simulink model "MC_PB_ESS3"  (Simulink 3.00)
settings: Solver=ode1  SolverMode=SingleTasking  StartTime=0.0  StopTime=2  FixedStep=1  RelTol=1e-3  AbsTol=1e-6
values from neighbouring files (symbols this model uses):
  ess_init_soc = vinf.test.ess_init_soc.FUDS    [J17_FUDS.m]    (also in J17_HFEDS.m = vinf.test.ess_init_soc.HWFET; J17_SC03.m = vinf.test.ess_init_soc.SC03; J17_UDDS.m = vinf.test.ess_init_soc.UDDS; J17_US06.m = vinf.test.ess_init_soc.US06)
undefined symbols (not defined in the file or in its folder): acc_elec_eff, acc_elec_pwr, ess_coulombic_eff, ess_max_ah_cap, ess_max_volts, ess_min_volts, ess_module_num, ess_on, ess_soc_current, ess_tmp, mc_inertia, mc_inpwr_map, mc_map_spd, mc_map_trq, mc_max_crrnt, mc_max_trq, mc_min_volts, mc_overtrq_factor, mc_spd_scale, mc_trq_scale, Tess, Tm, wm
settings Model: LastModifiedBy=vjohnson

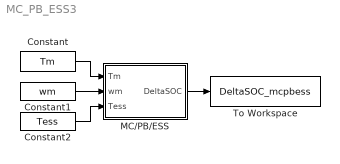
== system MC_PB_ESS3 ==
  Constant : Constant  Value=Tm
  Constant1 : Constant  Value=wm
  Constant2 : Constant  Value=Tess
  MC/PB/ESS : Subsystem
  To Workspace : ToWorkspace  VariableName=DeltaSOC_mcpbess  SampleTime=-1  SaveFormat=Matrix
  wires:
  Constant/1 -> MC/PB/ESS/1(Tm)
  Constant1/1 -> MC/PB/ESS/2(wm)
  MC/PB/ESS/1(DeltaSOC) -> To Workspace/1
  Constant2/1 -> MC/PB/ESS/3(Tess)

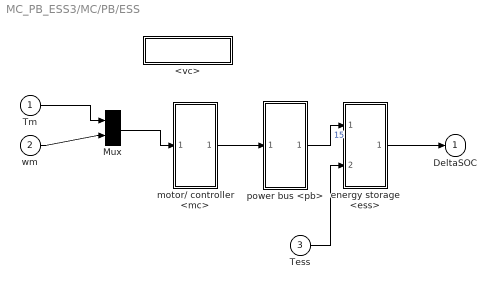
== system MC_PB_ESS3/MC/PB/ESS ==
  Tm : Inport  Port=1  PortWidth=-1  SampleTime=-1  DataType=auto
      settings: SignalType=auto
  wm : Inport  Port=2  PortWidth=-1  SampleTime=-1  DataType=auto
      settings: SignalType=auto
  Tess : Inport  Port=3  PortWidth=-1  SampleTime=-1  DataType=auto
      settings: SignalType=auto
  <vc> : Subsystem
      mask Display: disp('vehicle controls')
  Mux : Mux  Inputs=2
      settings: DisplayOption=none
  energy storage <ess> : Subsystem
  motor/ controller <mc> : Subsystem
  power bus <pb> : Subsystem
  DeltaSOC : Outport  Port=1  InitialOutput=0
  wires:
  Tm/1 -> Mux/1
  wm/1 -> Mux/2
  Mux/1 -> motor/ controller <mc>/1("torque and speed  req'd at rotor (Nm), (rad/s)")
  energy storage <ess>/1(delta SOC) -> DeltaSOC/1
  Tess/1 -> energy storage <ess>/2(Tess)
  power bus <pb>/1(power req'd from energy storage (W)) -> energy storage <ess>/1(power req'd into bus (W))  "15"
  motor/ controller <mc>/1(req'd motor input power (W)) -> power bus <pb>/1(req'd power output (W))

== system MC_PB_ESS3/MC/PB/ESS/<vc> ==
  motor controller logic : Subsystem
  shifting : Constant  Orientation=left  Value=0
  tag scope: P_mc_in_r=global
  wires:
  motor controller logic/1(req'd input power (W)1) -> [P_mc_in_r]
  [w_mc_out_r] -> motor controller logic/3(req'd output spd (rad/s))
  [P_mc_in_1lim] -> motor controller logic/2(req'd input power (W))
  [bus_voltage] -> motor controller logic/1(bus voltage)
  shifting/1 -> motor controller logic/4(shifting)

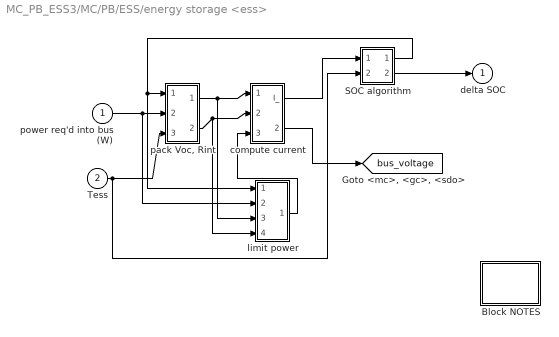
== system MC_PB_ESS3/MC/PB/ESS/energy storage <ess> ==
  power req'd into bus (W) : Inport  Port=1  PortWidth=-1  SampleTime=-1  DataType=auto
      settings: SignalType=auto
  Tess : Inport  Port=2  PortWidth=-1  SampleTime=-1  DataType=auto
      settings: SignalType=auto
  Block NOTES : Subsystem
      mask Display: disp('Block\nNOTES')
  SOC algorithm : Subsystem
  compute current : Subsystem
  limit power : Subsystem
  "pack Voc, Rint" : Subsystem
  delta SOC : Outport  Port=1  InitialOutput=0
  tag scope: bus_voltage=global
  wires:
  "pack Voc, Rint"/2(pack resistance) -> compute current/2(Rint), limit power/4(Rint)
  "pack Voc, Rint"/1(pack open- circuit voltage) -> compute current/1(Voc), limit power/3(Voc)
  SOC algorithm/1(SOC1) -> "pack Voc, Rint"/1(SOC (prev)), limit power/1(SOC)
  Tess/1 -> "pack Voc, Rint"/3(mod tmp   (C)), SOC algorithm/2(tmp (C))
  power req'd into bus (W)/1 -> "pack Voc, Rint"/2(req'd battery power (W)), limit power/2(Pbty)
  SOC algorithm/2(DeltaSOC) -> delta SOC/1
  compute current/2(V_) -> [bus_voltage]
  compute current/1(I_) -> SOC algorithm/1((A))
  limit power/1("Pbty, limited") -> compute current/3(limited output power (W))

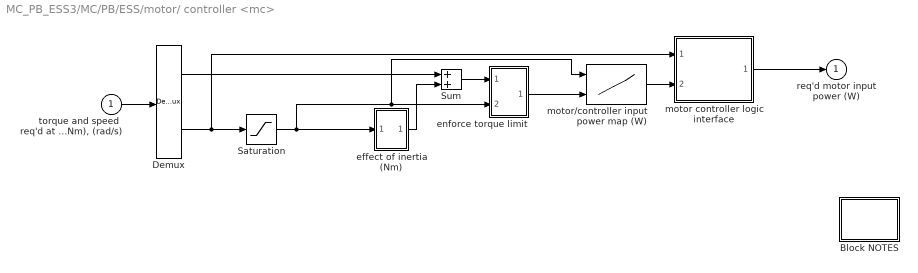
== system MC_PB_ESS3/MC/PB/ESS/motor/ controller <mc> ==
  "torque and speed  req'd at rotor (Nm), (rad/s)" : Inport  Port=1  PortWidth=-1  SampleTime=-1  DataType=auto
      settings: SignalType=auto
  Block NOTES : Subsystem
      mask Display: disp('Block\nNOTES')
  Demux : Demux  Outputs=2
  Saturation : Saturate  UpperLimit=max(mc_map_spd)*mc_spd_scale  LowerLimit=0
  Sum : Sum  Inputs=++  SaturateOnIntegerOverflow=on
  effect of inertia (Nm) : Subsystem
  enforce torque limit : Subsystem
  motor controller logic interface : Subsystem
  motor/controller input power map (W) : Lookup2D  RowIndex=mc_map_spd*mc_spd_scale  ColumnIndex=mc_map_trq*mc_trq_scale  OutputValues=mc_inpwr_map*mc_spd_scale*mc_trq_scale
  req'd motor input power (W) : Outport  Port=1  InitialOutput=0
  wires:
  Saturation/1 -> effect of inertia (Nm)/1(mc_spd_out_a), motor/controller input power map (W)/1, enforce torque limit/2(limited motor speed (rad/s))
  Sum/1 -> enforce torque limit/1(req'd motor torque (Nm))
  Demux/2 -> motor controller logic interface/1(w_mc_out_r), Saturation/1
  "torque and speed  req'd at rotor (Nm), (rad/s)"/1 -> Demux/1
  motor controller logic interface/1(P_mc_in_r) -> req'd motor input power (W)/1
  effect of inertia (Nm)/1(out_1) -> Sum/2
  motor/controller input power map (W)/1 -> motor controller logic interface/2(P_mc_in_1lim)
  enforce torque limit/1(limited motor torque (Nm)) -> motor/controller input power map (W)/2
  Demux/1 -> Sum/1

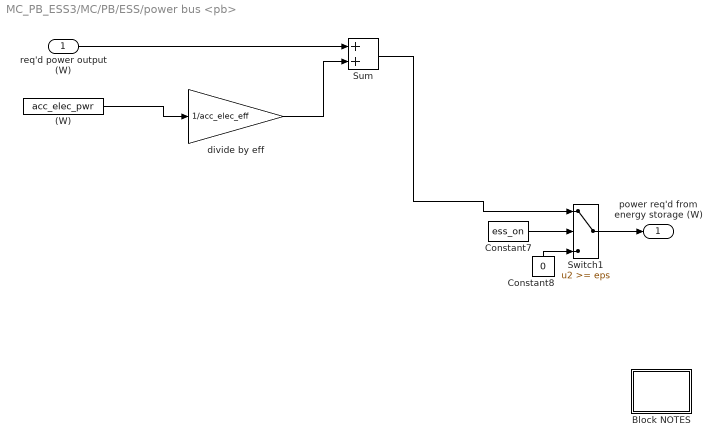
== system MC_PB_ESS3/MC/PB/ESS/power bus <pb> ==
  req'd power output (W) : Inport  Port=1  PortWidth=-1  SampleTime=-1  DataType=auto
      settings: SignalType=auto
  (W) : Constant  Value=acc_elec_pwr
  Block NOTES : Subsystem
      mask Display: disp('Block\nNOTES')
  Constant7 : Constant  Value=ess_on
  Constant8 : Constant  Orientation=up  Value=0
  Sum : Sum  Inputs=++  SaturateOnIntegerOverflow=on
  Switch1 : Switch  Threshold=eps
  divide by eff : Gain  Gain=1/acc_elec_eff  SaturateOnIntegerOverflow=on
  power req'd from energy storage (W) : Outport  Port=1
  wires:
  Constant8/1 -> Switch1/3
  Constant7/1 -> Switch1/2
  Switch1/1 -> power req'd from energy storage (W)/1
  req'd power output (W)/1 -> Sum/1
  divide by eff/1 -> Sum/2
  (W)/1 -> divide by eff/1
  Sum/1 -> Switch1/1

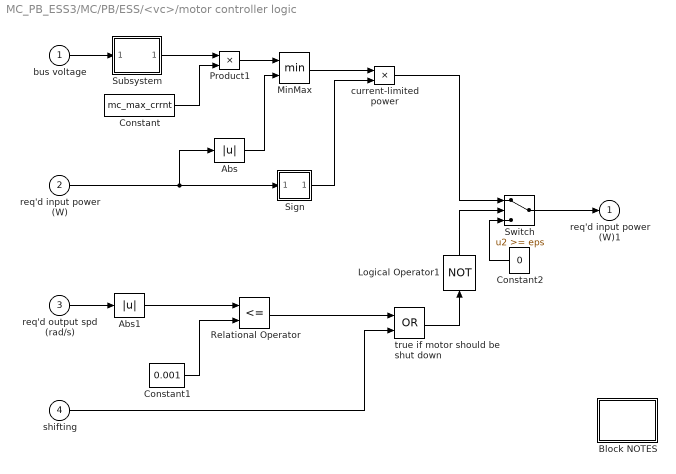
== system MC_PB_ESS3/MC/PB/ESS/<vc>/motor controller logic ==
  bus voltage : Inport  Port=1  PortWidth=-1  SampleTime=-1  DataType=auto
      settings: SignalType=auto
  req'd input power (W) : Inport  Port=2  PortWidth=-1  SampleTime=-1  DataType=auto
      settings: SignalType=auto
  req'd output spd (rad/s) : Inport  Port=3  PortWidth=-1  SampleTime=-1  DataType=auto
      settings: SignalType=auto
  shifting : Inport  Port=4  PortWidth=-1  SampleTime=-1  DataType=auto
      settings: SignalType=auto
  Abs : Abs
  Abs1 : Abs
  Block NOTES : Subsystem
      mask Display: disp('Block\nNOTES')
  Constant : Constant  Value=mc_max_crrnt
  Constant1 : Constant  Value=0.001
  Constant2 : Constant  Orientation=left  Value=0
  Logical Operator1 : Logic  Orientation=up  Operator=NOT  Inputs=1
  MinMax : MinMax  Function=min  Inputs=2
  Product1 : Product  Inputs=2  SaturateOnIntegerOverflow=on
  Relational Operator : RelationalOperator  Operator=<=
  Sign : Subsystem
      mask Type: Sign
      mask Description: y = sign(x)
      mask Help: Sign Function:\n\t\t\ty = 1 if x > 0\n\t\t\ty = 0 if x = 0\n\t\t\ty = -1 if x < 0
      mask Display: plot(-50,-50,50,50,[-50,50],[0,0],[0,0],[-50,50],[-40,0],[-30,-30],[0,40],[30,30])
  Subsystem : Subsystem  mask(Running Average){@1=2}
      mask prompts: @1 "Averaging Time (s)"
      mask help: Running Average
      mask init:
      | n=@1;
      mask Help: Output is the average of the last (Averaging Time) seconds of input.
      mask Display: disp('Running\nAverage')
  Switch : Switch  Threshold=eps
  current-limited power : Product  Inputs=2  SaturateOnIntegerOverflow=on
  true if motor should be shut down : Logic  Operator=OR  Inputs=2
  req'd input power (W)1 : Outport  Port=1  InitialOutput=0
  wires:
  shifting/1 -> true if motor should be shut down/2
  Logical Operator1/1 -> Switch/2
  true if motor should be shut down/1 -> Logical Operator1/1
  Subsystem/1(out_1) -> Product1/1
  bus voltage/1 -> Subsystem/1(in_1)
  Constant/1 -> Product1/2
  req'd input power (W)/1 -> Abs/1, Sign/1(in_1)
  Abs/1 -> MinMax/2
  Sign/1(out_1) -> current-limited power/2
  Constant2/1 -> Switch/3
  Switch/1 -> req'd input power (W)1/1
  current-limited power/1 -> Switch/1
  Relational Operator/1 -> true if motor should be shut down/1
  Constant1/1 -> Relational Operator/2
  req'd output spd (rad/s)/1 -> Abs1/1
  Abs1/1 -> Relational Operator/1
  MinMax/1 -> current-limited power/1
  Product1/1 -> MinMax/1

== system MC_PB_ESS3/MC/PB/ESS/energy storage <ess>/Block NOTES ==
  note: This block models the energy storage system as an SOC-dependent voltage
      | in series with an SOC- and current direction-dependent internal resistance.
      | SOC is computed assuming that A-h capacity is constant, but limited
      | such that a minimum voltage is never exceeded (replacing the
      | previous Peukert relationship which underpredicted battery capacity).
      |
      | Discharge power is limited here so as not to bring the bus (battery pack) voltage below
      | the minimum controller voltage or the minimum battery voltage and so as to allow
      | the solution of the quadratic eq'n for discharge current.
      |
      | Charge current is limited to ensure the voltage does not exceed a maximum
      | voltage
      |
      | Positive current is discharge current in the convention used here.
      | Power loss is computed as I*R+losses due to Coulombic (in)efficiency.
      |
      | Thermal modeling of the battery performance is modeled in the
      | OCV, Rint, and capacity.

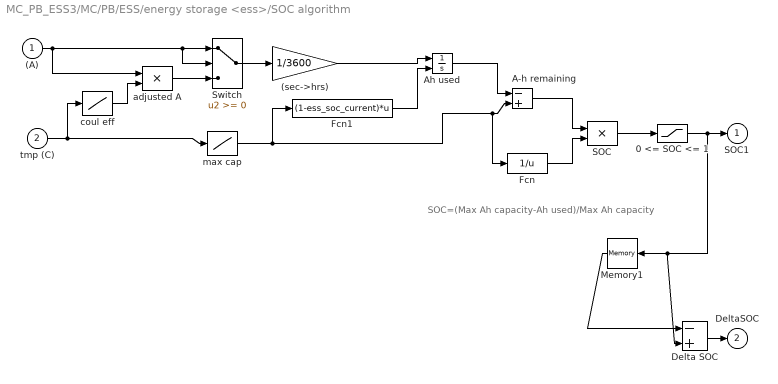
== system MC_PB_ESS3/MC/PB/ESS/energy storage <ess>/SOC algorithm ==
  note: SOC=(Max Ah capacity-Ah used)/Max Ah capacity
  (A) : Inport  Port=1  PortWidth=-1  SampleTime=-1  DataType=auto
      settings: SignalType=auto
  tmp (C) : Inport  Port=2  PortWidth=-1  SampleTime=-1  DataType=auto
      settings: SignalType=auto
  (sec->hrs) : Gain  Gain=1/3600  SaturateOnIntegerOverflow=on
  0 <= SOC <= 1 : Saturate  UpperLimit=1  LowerLimit=0
  A-h remaining : Sum  Inputs=-+  SaturateOnIntegerOverflow=on
  Ah used : Integrator  ExternalReset=none  InitialConditionSource=external  InitialCondition=(1-ess_init_soc)*ess_max_ah_cap  LimitOutput=off  UpperSaturationLimit=inf  LowerSaturationLimit=-inf  ShowSaturationPort=off  ShowStatePort=off  AbsoluteTolerance=auto
  Delta SOC : Sum  Inputs=-+  SaturateOnIntegerOverflow=on
  Fcn : Fcn  Expr=1/u
  Fcn1 : Fcn  Expr=(1-ess_soc_current)*u
  Memory1 : Memory  Orientation=left  X0=ess_soc_current(end)  InheritSampleTime=off
  SOC : Product  Inputs=2  SaturateOnIntegerOverflow=on
  Switch : Switch  Threshold=0
  adjusted A : Product  Inputs=2  SaturateOnIntegerOverflow=on
  coul eff : Lookup  InputValues=ess_tmp  OutputValues=ess_coulombic_eff
  max cap : Lookup  InputValues=ess_tmp  OutputValues=ess_max_ah_cap
  SOC1 : Outport  Port=1  InitialOutput=0
  DeltaSOC : Outport  Port=2  InitialOutput=ess_init_soc
  wires:
  (A)/1 -> Switch/2, Switch/1, adjusted A/1
  Switch/1 -> (sec->hrs)/1
  Ah used/1 -> A-h remaining/1
  Fcn/1 -> SOC/2
  SOC/1 -> 0 <= SOC <= 1/1
  A-h remaining/1 -> SOC/1
  tmp (C)/1 -> max cap/1, coul eff/1
  coul eff/1 -> adjusted A/2
  adjusted A/1 -> Switch/3
  max cap/1 -> A-h remaining/2, Fcn/1, Fcn1/1
  Fcn1/1 -> Ah used/2
  Delta SOC/1 -> DeltaSOC/1
  Memory1/1 -> Delta SOC/1
  0 <= SOC <= 1/1 -> SOC1/1, Memory1/1, Delta SOC/2
  (sec->hrs)/1 -> Ah used/1

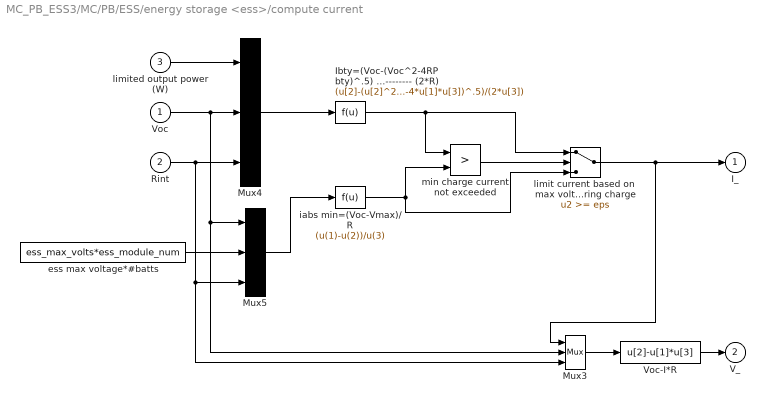
== system MC_PB_ESS3/MC/PB/ESS/energy storage <ess>/compute current ==
  Voc : Inport  Port=1  PortWidth=-1  SampleTime=-1  DataType=auto
      settings: SignalType=auto
  Rint : Inport  Port=2  PortWidth=-1  SampleTime=-1  DataType=auto
      settings: SignalType=auto
  limited output power (W) : Inport  Port=3  PortWidth=-1  SampleTime=-1  DataType=auto
      settings: SignalType=auto
  Ibty=(Voc-(Voc^2-4RPbty)^.5)        ----------------------------- (2*R) : Fcn  Expr=(u[2]-(u[2]^2-4*u[1]*u[3])^.5)/(2*u[3])
  Mux3 : Mux  Inputs=3
      settings: DisplayOption=none
  Mux4 : Mux  Inputs=3
      settings: DisplayOption=none
  Mux5 : Mux  Inputs=3
      settings: DisplayOption=none
  Voc-I*R : Fcn  Expr=u[2]-u[1]*u[3]
  ess max voltage*#batts : Constant  Value=ess_max_volts*ess_module_num
  iabs min=(Voc-Vmax)/R : Fcn  Expr=(u(1)-u(2))/u(3)
  limit current based on  max voltage during charge : Switch  Threshold=eps
  min charge current not exceeded : RelationalOperator  Operator=>
  I_ : Outport  Port=1  InitialOutput=0
  V_ : Outport  Port=2  InitialOutput=0
  wires:
  limited output power (W)/1 -> Mux4/1
  Voc/1 -> Mux4/2, Mux3/2, Mux5/1
  Rint/1 -> Mux4/3, Mux3/3, Mux5/3
  Ibty=(Voc-(Voc^2-4RPbty)^.5)        ----------------------------- (2*R)/1 -> min charge current not exceeded/1, limit current based on  max voltage during charge/1
  iabs min=(Voc-Vmax)/R/1 -> min charge current not exceeded/2, limit current based on  max voltage during charge/3
  limit current based on  max voltage during charge/1 -> I_/1, Mux3/1
  Mux3/1 -> Voc-I*R/1
  Mux4/1 -> Ibty=(Voc-(Voc^2-4RPbty)^.5)        ----------------------------- (2*R)/1
  Mux5/1 -> iabs min=(Voc-Vmax)/R/1
  ess max voltage*#batts/1 -> Mux5/2
  Voc-I*R/1 -> V_/1
  min charge current not exceeded/1 -> limit current based on  max voltage during charge/2

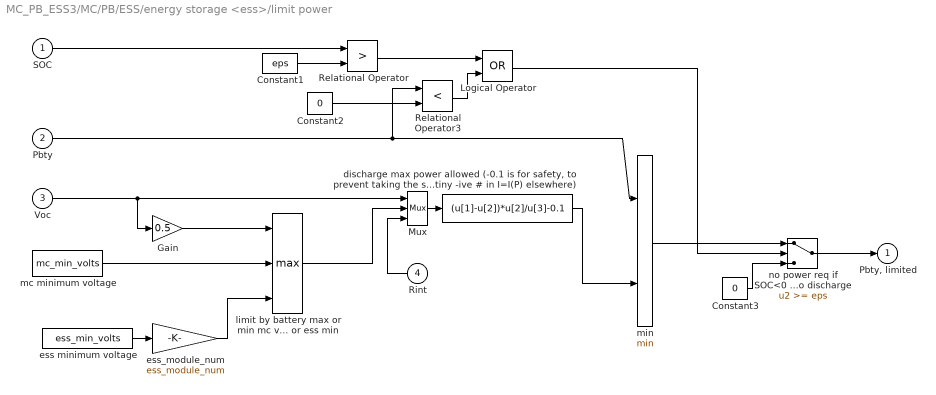
== system MC_PB_ESS3/MC/PB/ESS/energy storage <ess>/limit power ==
  SOC : Inport  Port=1  PortWidth=-1  SampleTime=-1  DataType=auto
      settings: SignalType=auto
  Pbty : Inport  Port=2  PortWidth=-1  SampleTime=-1  DataType=auto
      settings: SignalType=auto
  Voc : Inport  Port=3  PortWidth=-1  SampleTime=-1  DataType=auto
      settings: SignalType=auto
  Rint : Inport  Orientation=left  Port=4  PortWidth=-1  SampleTime=-1  DataType=auto
      settings: SignalType=auto
  Constant1 : Constant  Value=eps
  Constant2 : Constant  Value=0
  Constant3 : Constant  Value=0
  Gain : Gain  Gain=0.5  SaturateOnIntegerOverflow=on
  Logical Operator : Logic  Operator=OR  Inputs=2
  Mux : Mux  Inputs=3
      settings: DisplayOption=none
  Relational Operator : RelationalOperator  Operator=>
  Relational Operator3 : RelationalOperator  Operator=<
  "discharge max power allowed (-0.1 is for safety, to prevent taking the square of a tiny -ive # in I=I(P) elsewhere)" : Fcn  Expr=(u[1]-u[2])*u[2]/u[3]-0.1
  ess minimum voltage : Constant  Value=ess_min_volts
  ess_module_num : Gain  Gain=ess_module_num  SaturateOnIntegerOverflow=on
  limit by battery max or min mc voltage or ess min : MinMax  Function=max  Inputs=3
  mc minimum voltage : Constant  Value=mc_min_volts
  min : MinMax  Function=min  Inputs=2
  no power req if SOC<0 and trying  to discharge : Switch  Threshold=eps
  "Pbty, limited" : Outport  Port=1  InitialOutput=0
  wires:
  SOC/1 -> Relational Operator/1
  Constant1/1 -> Relational Operator/2
  Relational Operator/1 -> Logical Operator/1
  Pbty/1 -> Relational Operator3/1, min/1
  Constant2/1 -> Relational Operator3/2
  Relational Operator3/1 -> Logical Operator/2
  Constant3/1 -> no power req if SOC<0 and trying  to discharge/3
  no power req if SOC<0 and trying  to discharge/1 -> "Pbty, limited"/1
  Voc/1 -> Mux/1, Gain/1
  Mux/1 -> "discharge max power allowed (-0.1 is for safety, to prevent taking the square of a tiny -ive # in I=I(P) elsewhere)"/1
  Rint/1 -> Mux/3
  ess minimum voltage/1 -> ess_module_num/1
  ess_module_num/1 -> limit by battery max or min mc voltage or ess min/3
  Gain/1 -> limit by battery max or min mc voltage or ess min/1
  mc minimum voltage/1 -> limit by battery max or min mc voltage or ess min/2
  "discharge max power allowed (-0.1 is for safety, to prevent taking the square of a tiny -ive # in I=I(P) elsewhere)"/1 -> min/2
  limit by battery max or min mc voltage or ess min/1 -> Mux/2
  Logical Operator/1 -> no power req if SOC<0 and trying  to discharge/2
  min/1 -> no power req if SOC<0 and trying  to discharge/1

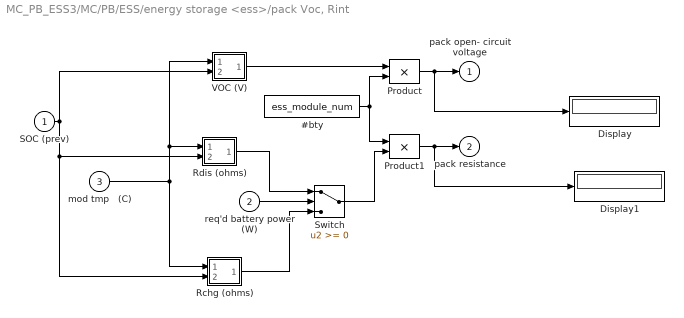
== system MC_PB_ESS3/MC/PB/ESS/energy storage <ess>/pack Voc, Rint ==
  SOC (prev) : Inport  Port=1  PortWidth=-1  SampleTime=-1  DataType=auto
      settings: SignalType=auto
  req'd battery power (W) : Inport  Port=2  PortWidth=-1  SampleTime=-1  DataType=auto
      settings: SignalType=auto
  mod tmp   (C) : Inport  Port=3  PortWidth=-1  SampleTime=-1  DataType=auto
      settings: SignalType=auto
  #bty : Constant  Value=ess_module_num
  Display : Display
      settings: Format=short
  Display1 : Display
      settings: Format=short
  Product : Product  Inputs=2  SaturateOnIntegerOverflow=on
  Product1 : Product  Inputs=2  SaturateOnIntegerOverflow=on
  Rchg (ohms) : Subsystem  mask(2-D Table Lookup){@1=ess_tmp, @2=ess_soc, @3=ess_r_chg}
      mask prompts: @1 "X Index"; @2 "Y Index"; @3 "Table"
      mask help:
      | Two Dimensional Table Lookup
      | The first input corresponds to X Index and the second input corresponds to the Y Index
      mask init:
      | xindex=@1; yindex=@2; table=@3; sftab2chk(xindex,yindex,table);
      mask Help: This block returns a linearly interpolated intersection from the table using the X index (which corresponds to the rows of the table) and the Y index (which corresponds to the columns of the table).  Extrapolation is used.
      mask Display: plot(-10,-10,110,110,[90,50,10],[90,40,30],[90,50,10],[50,26,20],[90,50,10],[22,13,10])
  Rdis (ohms) : Subsystem  mask(2-D Table Lookup){@1=ess_tmp, @2=ess_soc, @3=ess_r_dis}
      mask prompts: @1 "X Index"; @2 "Y Index"; @3 "Table"
      mask help:
      | Two Dimensional Table Lookup
      | The first input corresponds to X Index and the second input corresponds to the Y Index
      mask init:
      | xindex=@1; yindex=@2; table=@3; sftab2chk(xindex,yindex,table);
      mask Help: This block returns a linearly interpolated intersection from the table using the X index (which corresponds to the rows of the table) and the Y index (which corresponds to the columns of the table).  Extrapolation is used.
      mask Display: plot(-10,-10,110,110,[90,50,10],[90,40,30],[90,50,10],[50,26,20],[90,50,10],[22,13,10])
  Switch : Switch  Threshold=0
  VOC (V) : Subsystem  mask(2-D Table Lookup){@1=ess_tmp, @2=ess_soc, @3=ess_voc}
      mask prompts: @1 "X Index"; @2 "Y Index"; @3 "Table"
      mask help:
      | Two Dimensional Table Lookup
      | The first input corresponds to X Index and the second input corresponds to the Y Index
      mask init:
      | xindex=@1; yindex=@2; table=@3; sftab2chk(xindex,yindex,table);
      mask Help: This block returns a linearly interpolated intersection from the table using the X index (which corresponds to the rows of the table) and the Y index (which corresponds to the columns of the table).  Extrapolation is used.
      mask Display: plot(-10,-10,110,110,[90,50,10],[90,40,30],[90,50,10],[50,26,20],[90,50,10],[22,13,10])
  pack open- circuit voltage : Outport  Port=1  InitialOutput=0
  pack resistance : Outport  Port=2  InitialOutput=0
  wires:
  #bty/1 -> Product1/1, Product/2
  VOC (V)/1(table out) -> Product/1
  Rchg (ohms)/1(table out) -> Switch/3
  Rdis (ohms)/1(table out) -> Switch/1
  req'd battery power (W)/1 -> Switch/2
  Switch/1 -> Product1/2
  SOC (prev)/1 -> VOC (V)/2(y0), Rdis (ohms)/2(y0), Rchg (ohms)/2(y0)
  mod tmp   (C)/1 -> VOC (V)/1(x0), Rdis (ohms)/1(x0), Rchg (ohms)/1(x0)
  Product/1 -> pack open- circuit voltage/1, Display/1
  Product1/1 -> pack resistance/1, Display1/1

== system MC_PB_ESS3/MC/PB/ESS/motor/ controller <mc>/Block NOTES ==
  note: Available torque is computed from available power by assuming that the ratio of rotor torque to input
      | (electric) power is the same for the actual/achievable situation as was computed for the request.  This
      | is mathematically equivalent to assuming that the motor/controller efficiency.  Rotor speed for the
      | actual/achievable calculations is as computed in the 'request' branch.
  note: This motor/controller model includes loss data, rotational inertia, and performance limits.

== system MC_PB_ESS3/MC/PB/ESS/motor/ controller <mc>/effect of inertia (Nm) ==
  mc_spd_out_a : Inport  Port=1  PortWidth=-1  SampleTime=-1  DataType=auto
      settings: SignalType=auto
  Gain : Gain  Gain=mc_inertia  SaturateOnIntegerOverflow=on
  alpha : Derivative
  out_1 : Outport  Port=1  InitialOutput=0
  wires:
  alpha/1 -> Gain/1
  mc_spd_out_a/1 -> alpha/1
  Gain/1 -> out_1/1

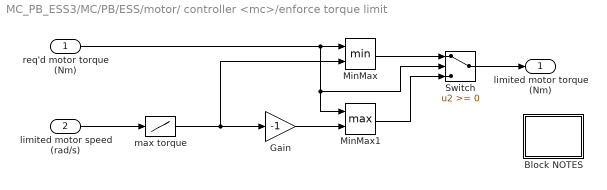
== system MC_PB_ESS3/MC/PB/ESS/motor/ controller <mc>/enforce torque limit ==
  req'd motor torque (Nm) : Inport  Port=1  PortWidth=-1  SampleTime=-1  DataType=auto
      settings: SignalType=auto
  limited motor speed (rad/s) : Inport  Port=2  PortWidth=-1  SampleTime=-1  DataType=auto
      settings: SignalType=auto
  Block NOTES : Subsystem
      mask Display: disp('Block\nNOTES')
  Gain : Gain  Gain=-1  SaturateOnIntegerOverflow=on
  MinMax : MinMax  Function=min  Inputs=2
  MinMax1 : MinMax  Function=max  Inputs=2
  Switch : Switch  Threshold=0
  max torque : Lookup  InputValues=mc_map_spd*mc_spd_scale  OutputValues=mc_max_trq*mc_overtrq_factor*mc_trq_scale
  limited motor torque (Nm) : Outport  Port=1
  wires:
  limited motor speed (rad/s)/1 -> max torque/1
  Gain/1 -> MinMax1/2
  MinMax1/1 -> Switch/3
  MinMax/1 -> Switch/1
  Switch/1 -> limited motor torque (Nm)/1
  req'd motor torque (Nm)/1 -> Switch/2, MinMax1/1, MinMax/1
  max torque/1 -> Gain/1, MinMax/2

== system MC_PB_ESS3/MC/PB/ESS/motor/ controller <mc>/motor controller logic interface ==
  w_mc_out_r : Inport  Port=1  PortWidth=-1  SampleTime=-1  DataType=auto
      settings: SignalType=auto
  P_mc_in_1lim : Inport  Port=2  PortWidth=-1  SampleTime=-1  DataType=auto
      settings: SignalType=auto
  P_mc_in_r : Outport  Port=1  InitialOutput=0
  tag scope: P_mc_in_1lim=global, w_mc_out_r=global
  wires:
  [P_mc_in_r] -> P_mc_in_r/1
  w_mc_out_r/1 -> [w_mc_out_r]
  P_mc_in_1lim/1 -> [P_mc_in_1lim]

== system MC_PB_ESS3/MC/PB/ESS/power bus <pb>/Block NOTES ==
  note: This power bus requires power from (or distributes power to)
      | the generator first, taking the balance from the energy
      | storage system.

== system MC_PB_ESS3/MC/PB/ESS/<vc>/motor controller logic/Block NOTES ==
  note: This block models a motor/controller's logic, modulating the power input requirement as follows:
      | - enforcing the maximum current limit of the motor/controller
      | - shutting the motor off if the average speed over the time step ==0
      | - shutting the motor off if the transmission is shifting.

== system MC_PB_ESS3/MC/PB/ESS/<vc>/motor controller logic/Sign ==
  in_1 : Inport  Port=1  PortWidth=-1  SampleTime=-1  DataType=auto
      settings: SignalType=auto
  Constant : Constant  Value=0
  Relational Operator : RelationalOperator  Operator=>
  Relational Operator1 : RelationalOperator  Operator=<
  Sum : Sum  Inputs=+-  SaturateOnIntegerOverflow=on
  out_1 : Outport  Port=1  InitialOutput=0
  wires:
  Sum/1 -> out_1/1
  Relational Operator/1 -> Sum/1
  Relational Operator1/1 -> Sum/2
  Constant/1 -> Relational Operator/2, Relational Operator1/2
  in_1/1 -> Relational Operator1/1, Relational Operator/1

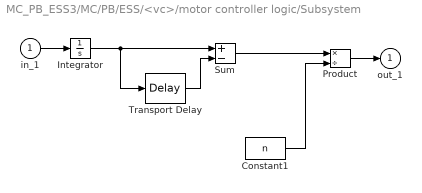
== system MC_PB_ESS3/MC/PB/ESS/<vc>/motor controller logic/Subsystem ==
  in_1 : Inport  Port=1  PortWidth=-1  SampleTime=-1  DataType=auto
      settings: SignalType=auto
  Constant1 : Constant  Value=n
  Integrator : Integrator  ExternalReset=none  InitialConditionSource=internal  InitialCondition=0  LimitOutput=off  UpperSaturationLimit=inf  LowerSaturationLimit=-inf  ShowSaturationPort=off  ShowStatePort=off  AbsoluteTolerance=auto
  Product : Product  Inputs=*/  SaturateOnIntegerOverflow=on
  Sum : Sum  Inputs=+-  SaturateOnIntegerOverflow=on
  Transport Delay : TransportDelay  DelayTime=n  InitialInput=0  BufferSize=1024
  out_1 : Outport  Port=1  InitialOutput=0
  wires:
  Integrator/1 -> Sum/1, Transport Delay/1
  Transport Delay/1 -> Sum/2
  Sum/1 -> Product/1
  in_1/1 -> Integrator/1
  Product/1 -> out_1/1
  Constant1/1 -> Product/2

== system MC_PB_ESS3/MC/PB/ESS/energy storage <ess>/pack Voc, Rint/Rchg (ohms) ==
  x0 : Inport  Port=1  PortWidth=-1  SampleTime=-1  DataType=auto
      settings: SignalType=auto
  y0 : Inport  Port=2  PortWidth=-1  SampleTime=-1  DataType=auto
      settings: SignalType=auto
  Mux : Mux  Inputs=2
      settings: DisplayOption=none
  S-function : S-Function  FunctionName=sftable2  Parameters=xindex, yindex, table  PortCounts=[]  SFunctionModules=''
  table out : Outport  Port=1  InitialOutput=0
  wires:
  y0/1 -> Mux/2
  S-function/1 -> table out/1
  x0/1 -> Mux/1
  Mux/1 -> S-function/1

== system MC_PB_ESS3/MC/PB/ESS/energy storage <ess>/pack Voc, Rint/Rdis (ohms) ==
  x0 : Inport  Port=1  PortWidth=-1  SampleTime=-1  DataType=auto
      settings: SignalType=auto
  y0 : Inport  Port=2  PortWidth=-1  SampleTime=-1  DataType=auto
      settings: SignalType=auto
  Mux : Mux  Inputs=2
      settings: DisplayOption=none
  S-function : S-Function  FunctionName=sftable2  Parameters=xindex, yindex, table  PortCounts=[]  SFunctionModules=''
  table out : Outport  Port=1  InitialOutput=0
  wires:
  y0/1 -> Mux/2
  S-function/1 -> table out/1
  x0/1 -> Mux/1
  Mux/1 -> S-function/1

== system MC_PB_ESS3/MC/PB/ESS/energy storage <ess>/pack Voc, Rint/VOC (V) ==
  x0 : Inport  Port=1  PortWidth=-1  SampleTime=-1  DataType=auto
      settings: SignalType=auto
  y0 : Inport  Port=2  PortWidth=-1  SampleTime=-1  DataType=auto
      settings: SignalType=auto
  Mux : Mux  Inputs=2
      settings: DisplayOption=none
  S-function : S-Function  FunctionName=sftable2  Parameters=xindex, yindex, table  PortCounts=[]  SFunctionModules=''
  table out : Outport  Port=1  InitialOutput=0
  wires:
  y0/1 -> Mux/2
  S-function/1 -> table out/1
  x0/1 -> Mux/1
  Mux/1 -> S-function/1

== system MC_PB_ESS3/MC/PB/ESS/motor/ controller <mc>/enforce torque limit/Block NOTES ==
  note: This block enforces the maximum torque production and absorption
      | capability limits of the motor.  It assumes that exactly as much torque
      | can be absorbed as can be produced at a given speed.
